simulink model "Closed_Loop"  (R2016b)
settings: Solver=VariableStepAuto  StartTime=0.0  StopTime=40  RelTol=1e-3
settings Model: Creator=Yazdanpanah  LastModifiedBy=fatae
settings DataIOCC: ReturnWorkspaceOutputs=on
settings SFSimCC: SimUseLocalCustomCode=on
settings RTWCC: RTWUseLocalCustomCode=on

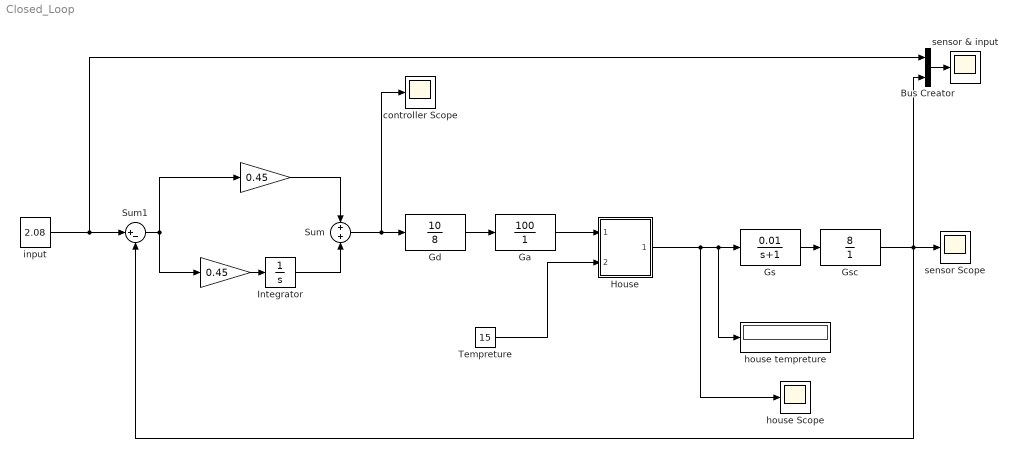
== system Closed_Loop ==
  " " : Gain  Gain=0.45
  " " : Gain  Gain=0.45
  Bus Creator : BusCreator  Inputs=2
  "Ga " : TransferFcn  Numerator=[100]  Denominator=[0 1]
  Gd : TransferFcn  Numerator=[10]  Denominator=[0 8]
  "Gs " : TransferFcn  Numerator=[0.01]  Denominator=[1 1]
  "Gsc " : TransferFcn  Numerator=[8]  Denominator=[0 1]
  House : Subsystem
      mask Display: image(fullfile(matlabroot,'toolbox','simulink','simdemos','simgeneral','images','HouseHeatHousePix.svg'))
  Integrator : Integrator
  Sum : Sum
  Sum1 : Sum  Inputs=|+-
  Tempreture : Constant  Value=15
  controller Scope : Scope
  house Scope : Scope
  house tempreture : Display
  "input " : Constant  Value=2.08
  sensor & input : Scope
  sensor Scope : Scope
  wires:
  Sum/1 -> controller Scope/1, Gd/1
  "Gsc "/1 -> Bus Creator/2, Sum1/2, sensor Scope/1
  Bus Creator/1 -> sensor & input/1
  Sum1/1 -> " "/1, " "/1
  Integrator/1 -> Sum/2
  " "/1 -> Integrator/1
  House/1(Room Temp Troom) -> "Gs "/1, house tempreture/1, house Scope/1
  Gd/1 -> "Ga "/1
  "Gs "/1 -> "Gsc "/1
  Tempreture/1 -> House/2(Outdoor Temp Tout)
  "input "/1 -> Bus Creator/1, Sum1/1
  "Ga "/1 -> House/1(Heater QDot In)
  " "/1 -> Sum/1

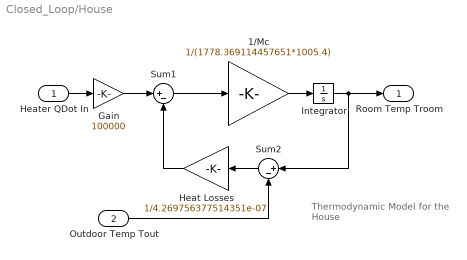
== system Closed_Loop/House ==
  note: Thermodynamic Model
      | for the House
  Heater QDot In : Inport
  Outdoor Temp Tout : Inport  Port=2
  1/Mc : Gain  Gain=1/(1778.369114457651*1005.4)  SaturateOnIntegerOverflow=on  OutDataTypeStr=Inherit: Same as input  ParamDataTypeStr=Inherit: Same as input
  Gain : Gain  Gain=100000
  Heat Losses : Gain  Gain=1/4.269756377514351e-07  SaturateOnIntegerOverflow=on  OutDataTypeStr=Inherit: Same as input  ParamDataTypeStr=Inherit: Same as input
  Integrator : Integrator  InitialCondition=20
  Sum1 : Sum  Inputs=|+-  SaturateOnIntegerOverflow=on  InputSameDT=on  OutDataTypeStr=Inherit: Same as first input
  Sum2 : Sum  Inputs=|+-  SaturateOnIntegerOverflow=on  InputSameDT=on  OutDataTypeStr=Inherit: Same as first input
  Room Temp Troom : Outport  InitialOutput=0
  wires:
  Outdoor Temp Tout/1 -> Sum2/2
  Heater QDot In/1 -> Gain/1
  Sum1/1 -> 1/Mc/1
  Sum2/1 -> Heat Losses/1
  Heat Losses/1 -> Sum1/2
  1/Mc/1 -> Integrator/1
  Integrator/1 -> Sum2/1, Room Temp Troom/1
  Gain/1 -> Sum1/1
